simulink model "Reg_Optim"  (R2017b)
settings: Solver=VariableStepAuto  StartTime=0.0  StopTime=60.0  RelTol=1e-3
values from neighbouring files (symbols this model uses):
  C = [0 1 0 0 0]    [Regul_Luenbergh.m]    (also in Regul_Luenbergh2.m; Regul_Modal.m; Regul_Modal2.m; Regul_Optim.m)
  iv = 2.2    [Regul_Luenbergh.m]    (also in Regul_Luenbergh2.m; Regul_Modal.m; Regul_Modal2.m; Regul_Optim.m)
  Kopt_m = -Kopt    [Regul_Optim.m]    (also in Regul_Optim2.m)
  Kopt_md = -Koptd    [Regul_Optim2.m]
  Tcn = 0.15    [Regul_Luenbergh.m]    (also in Regul_Luenbergh2.m; Regul_Modal.m; Regul_Modal2.m; Regul_Optim.m)
undefined symbols (not defined in the file or in its folder): Ad, Bd, Cd
settings Model: Creator=ASUS_302  LastModifiedBy=ASUS_302

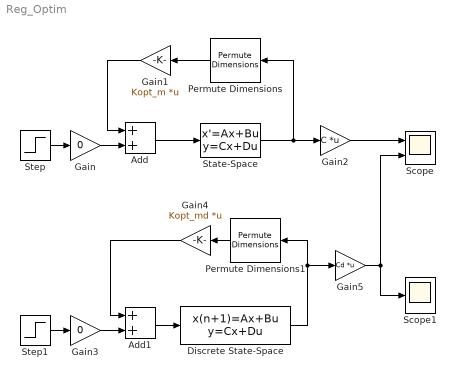
== system Reg_Optim ==
  Add : Sum
  Add1 : Sum
  Discrete State-Space : DiscreteStateSpace  A=Ad  B=Bd  C=eye(5)  D=zeros(5,1)  InitialCondition=[1;1;1;1;1]  SampleTime=0.1
  Gain : Gain  Gain=0
  Gain1 : Gain  Gain=Kopt_m  Multiplication=Matrix(K*u)
  Gain2 : Gain  Gain=C  Multiplication=Matrix(K*u)
  Gain3 : Gain  Gain=0
  Gain4 : Gain  Gain=Kopt_md  Multiplication=Matrix(K*u)
  Gain5 : Gain  Gain=Cd  Multiplication=Matrix(K*u)
  Permute Dimensions : PermuteDimensions
  Permute Dimensions1 : PermuteDimensions
  Scope : Scope  NumInputPorts=2
  Scope1 : Scope
  State-Space : StateSpace  A=|  B=[0; 0; 0; 0; iv/Tcn];  C=eye(5)  D=zeros(5,1)  InitialCondition=[1;1;1;1;1]
      | [c1 c2  0    c3      0;
      |    c4 c5  0    c6     c7;
      |    c8 c9  0    c10    c11;
      |     0  0  1    0       0;
      |     0  0 c12 iv/Tcn -1/Tcn];
  Step : Step  Time=0.01  SampleTime=0
  Step1 : Step  Time=0.01  SampleTime=0
  wires:
  Add/1 -> State-Space/1
  Step/1 -> Gain/1
  Gain2/1 -> Scope/1
  Permute Dimensions/1 -> Gain1/1
  Gain1/1 -> Add/1
  Gain/1 -> Add/2
  State-Space/1 -> Permute Dimensions/1, Gain2/1
  Step1/1 -> Gain3/1
  Gain4/1 -> Add1/1
  Add1/1 -> Discrete State-Space/1
  Gain3/1 -> Add1/2
  Gain5/1 -> Scope/2, Scope1/1
  Discrete State-Space/1 -> Gain5/1, Permute Dimensions1/1
  Permute Dimensions1/1 -> Gain4/1
